simulink model "sobel_filter"  (Simulink 7.9)
settings: Solver=ode45  StartTime=0.0  StopTime=180*320  RelTol=1e-3
undefined symbols (not defined in the file): gray
libraries: xbsIndex_r4 x48, dspsigattribs x5, visionsinks x3, visiongeotforms x3, visionsources x1
settings Model: Creator=COMPUTER  LastModifiedBy=COMPUTER

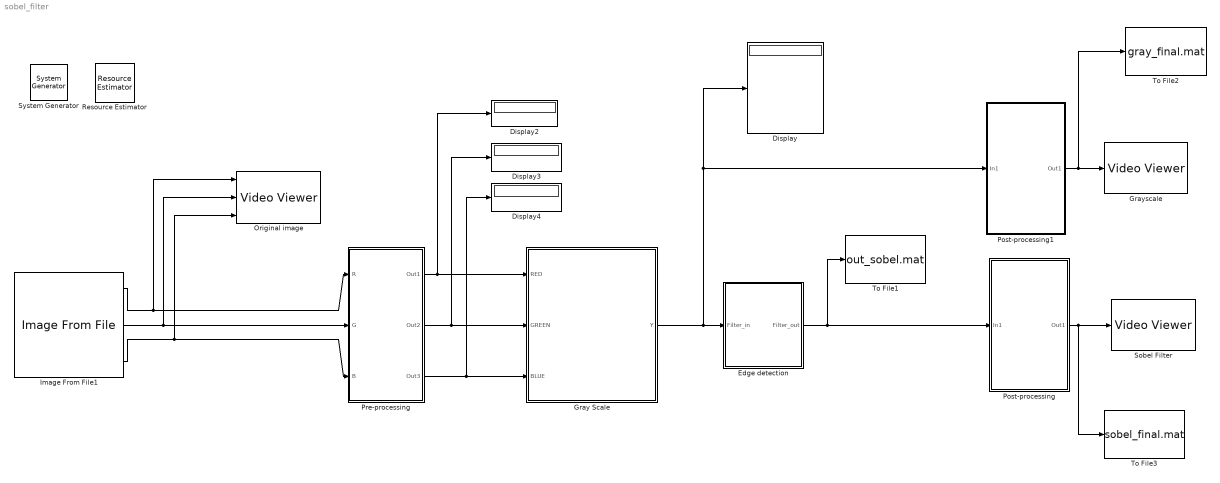
== system sobel_filter ==
  " System Generator" : xbsIndex_r4/ System Generator  Tag=genX  xilinxfamily=kintex7  part=xc7k325t  speed=-3  package=fbg676  synthesis_tool=XST  clock_wrapper=Clock Enables  directory=D:/DOAN1/Gray_conversion/ISE_software  proj_type=Project Navigator  Synth_file=XST Defaults  Impl_file=ISE Defaults  testbench=on  simulink_period=1  sysclk_period=10  dcm_input_clock_period=10  incr_netlist=off  trim_vbits=Everywhere in SubSystem  dbl_ovrd=According to Block Masks  core_generation=According to Block Masks  run_coregen=off  deprecated_control=off  eval_field=0  block_type=sysgen
  Display{,2..4} (4 alike) : Display
  Edge detection : Subsystem
  Gray Scale : Subsystem
  Grayscale : visionsinks/Video Viewer  inputType=Obsolete7b  imagePorts=One multidimensional signal  useColorMap=off  colormapValue=gray(256)  specRange=off  minInputVal=0  maxInputVal=255  FigPos=[2 1039 958 398]  AxisZoom=on  trueSizedOnce=off  OpenAtMdlStart=on
  Image From File1 : visionsources/Image From File  Tag=vipblks_nd  FileName=D:\DOAN1\Gray_conversion\hardware\straight_line_180_320.jpg  imagePorts=Separate color signals  Ts=inf  ImageDataType=uint8  Signed=on  WordLength=16  sdImageDataType=uint(8)  FractionLengthMode=User-defined  FractionLength=15  OutPortLabels=R|G|B
  Original image : visionsinks/Video Viewer  inputType=Obsolete7b  imagePorts=Separate color signals  useColorMap=off  colormapValue=gray(256)  specRange=off  minInputVal=0  maxInputVal=255  FigPos=[454 877 829 440]  AxisZoom=on  trueSizedOnce=off  OpenAtMdlStart=on
  Post-processing : Subsystem
  Post-processing1 : Subsystem
  Pre-processing : Subsystem
  Resource Estimator : xbsIndex_r4/Resource Estimator  Tag=resEstTag  Slices=0  FFs=0  BRAMs=0  LUTs=0  IOBs=0  EBMs=0  TBUFs=0  xl_use_estimator_area=off  est_options=Estimate  block_type=resource_estimator
      settings: AttributesFormatString=Resource\nEstimator
  Sobel Filter : visionsinks/Video Viewer  inputType=Obsolete7b  imagePorts=One multidimensional signal  useColorMap=off  colormapValue=gray(256)  specRange=off  minInputVal=0  maxInputVal=255  FigPos=[962 1039 958 919]  AxisZoom=on  trueSizedOnce=off  OpenAtMdlStart=on
  To File1 : ToFile  Filename=out_sobel.mat  MatrixName=sobel
  To File2 : ToFile  Filename=gray_final.mat  MatrixName=gray_final  SaveFormat=Timeseries
  To File3 : ToFile  Filename=sobel_final.mat  MatrixName=sobel_final  SaveFormat=Timeseries
  wires:
  Edge detection/1(Filter_out) -> Post-processing/1(In1), To File1/1
  Post-processing/1(Out1) -> Sobel Filter/1, To File3/1
  Pre-processing/1(Out1) -> Gray Scale/1(RED), Display2/1
  Image From File1/1 -> Original image/1, Pre-processing/1(R)
  Pre-processing/2(Out2) -> Gray Scale/2(GREEN), Display3/1
  Image From File1/2 -> Original image/2, Pre-processing/2(G)
  Pre-processing/3(Out3) -> Gray Scale/3(BLUE), Display4/1
  Image From File1/3 -> Original image/3, Pre-processing/3(B)
  Gray Scale/1(Y) -> Edge detection/1(Filter_in), Post-processing1/1(In1), Display/1
  Post-processing1/1(Out1) -> Grayscale/1, To File2/1

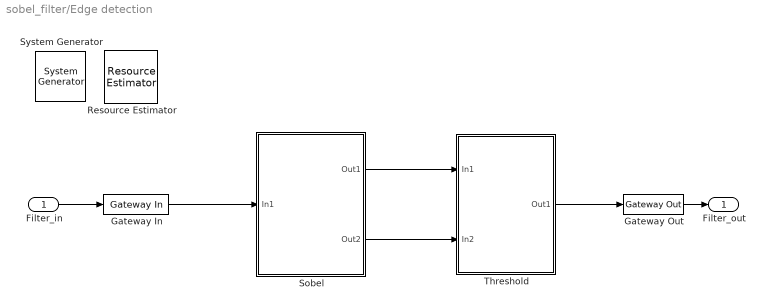
== system sobel_filter/Edge detection ==
  Filter_in : Inport
  " System Generator" : xbsIndex_r4/ System Generator  Tag=genX  xilinxfamily=kintex7  part=xc7k325t  speed=-3  package=fbg676  synthesis_tool=XST  clock_wrapper=Clock Enables  directory=./netlist  proj_type=Project Navigator  Synth_file=XST Defaults  Impl_file=ISE Defaults  testbench=off  simulink_period=1  sysclk_period=1.000000e+01  dcm_input_clock_period=10  incr_netlist=off  trim_vbits=Everywhere in SubSystem  dbl_ovrd=According to Block Masks  core_generation=According to Block Masks  run_coregen=off  deprecated_control=off  eval_field=0  block_type=sysgen
  Gateway In : xbsIndex_r4/Gateway In  gui_display_data_type=Fixed-point  arith_type=Unsigned  n_bits=8  bin_pt=0  preci_type=Single  exp_width=8  frac_width=24  quantization="Round  (unbiased: +/- Inf)"  overflow=Saturate  period=1  dbl_ovrd=off  timing_constraint=None  locs_specified=off  LOCs={}  UseAsADC=off  ADCChannel='1'  inherit_from_input=off  hdl_port=on  block_type=gatewayin
  Gateway Out : xbsIndex_r4/Gateway Out  inherit_from_input=off  hdl_port=on  timing_constraint="Data Rate;  Set 'FAST' Attribute"  locs_specified=off  LOCs={}  UseAsDAC=off  DACChannel='1'  block_type=gatewayout
  Resource Estimator : xbsIndex_r4/Resource Estimator  Tag=resEstTag  Slices=0  FFs=0  BRAMs=0  LUTs=0  IOBs=0  EBMs=0  TBUFs=0  xl_use_estimator_area=off  est_options=Estimate  block_type=resource_estimator
      settings: AttributesFormatString=Resource\nEstimator
  Sobel : Subsystem
  Threshold : Subsystem
  Filter_out : Outport
  wires:
  Filter_in/1 -> Gateway In/1
  Gateway Out/1 -> Filter_out/1
  Gateway In/1 -> Sobel/1(In1)
  Threshold/1(Out1) -> Gateway Out/1
  Sobel/1(Out1) -> Threshold/1(In1)
  Sobel/2(Out2) -> Threshold/2(In2)

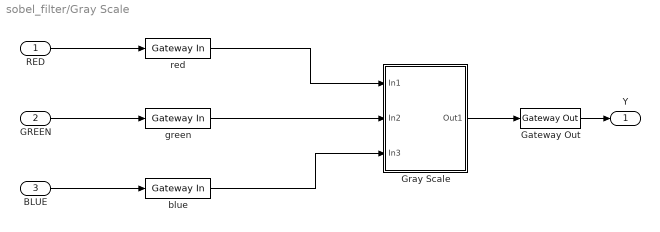
== system sobel_filter/Gray Scale ==
  RED : Inport
  GREEN : Inport  Port=2
  BLUE : Inport  Port=3
  Gateway Out : xbsIndex_r4/Gateway Out  inherit_from_input=off  hdl_port=on  timing_constraint="Data Rate;  Set 'FAST' Attribute"  locs_specified=off  LOCs={}  UseAsDAC=off  DACChannel='1'  block_type=gatewayout
  Gray Scale : Subsystem
  blue : xbsIndex_r4/Gateway In  gui_display_data_type=Fixed-point  arith_type="Signed  (2's comp)"  n_bits=8  bin_pt=0  preci_type=Single  exp_width=8  frac_width=24  quantization="Round  (unbiased: +/- Inf)"  overflow=Saturate  period=1  dbl_ovrd=off  timing_constraint=None  locs_specified=off  LOCs={}  UseAsADC=off  ADCChannel='1'  inherit_from_input=off  hdl_port=on  block_type=gatewayin
  green : xbsIndex_r4/Gateway In  gui_display_data_type=Fixed-point  arith_type="Signed  (2's comp)"  n_bits=8  bin_pt=0  preci_type=Single  exp_width=8  frac_width=24  quantization="Round  (unbiased: +/- Inf)"  overflow=Saturate  period=1  dbl_ovrd=off  timing_constraint=None  locs_specified=off  LOCs={}  UseAsADC=off  ADCChannel='1'  inherit_from_input=off  hdl_port=on  block_type=gatewayin
  red : xbsIndex_r4/Gateway In  gui_display_data_type=Fixed-point  arith_type=Unsigned  n_bits=8  bin_pt=0  preci_type=Single  exp_width=8  frac_width=24  quantization="Round  (unbiased: +/- Inf)"  overflow=Saturate  period=1  dbl_ovrd=off  timing_constraint=None  locs_specified=off  LOCs={}  UseAsADC=off  ADCChannel='1'  inherit_from_input=off  hdl_port=on  block_type=gatewayin
  Y : Outport
  wires:
  RED/1 -> red/1
  GREEN/1 -> green/1
  BLUE/1 -> blue/1
  Gateway Out/1 -> Y/1
  Gray Scale/1(Out1) -> Gateway Out/1
  red/1 -> Gray Scale/1(In1)
  green/1 -> Gray Scale/2(In2)
  blue/1 -> Gray Scale/3(In3)

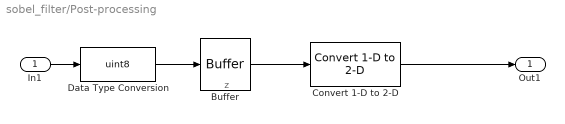
== system sobel_filter/Post-processing ==
  note: z
  In1 : Inport
  Buffer : Buffer  N=180*320
  Convert 1-D to 2-D : dspsigattribs/Convert 1-D to 2-D  M=180  N=320  frameBasedOut=off
  Data Type Conversion : DataTypeConversion  OutDataTypeStr=uint8  RndMeth=Round
  Out1 : Outport
  wires:
  Buffer/1 -> Convert 1-D to 2-D/1
  Convert 1-D to 2-D/1 -> Out1/1
  In1/1 -> Data Type Conversion/1
  Data Type Conversion/1 -> Buffer/1

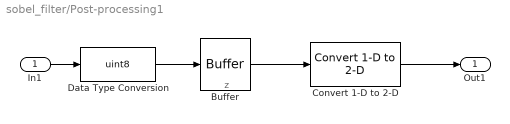
== system sobel_filter/Post-processing1 ==
  note: z
  In1 : Inport
  Buffer : Buffer  N=180*320
  Convert 1-D to 2-D : dspsigattribs/Convert 1-D to 2-D  M=180  N=320  frameBasedOut=off
  Data Type Conversion : DataTypeConversion  OutDataTypeStr=uint8
  Out1 : Outport
  wires:
  Buffer/1 -> Convert 1-D to 2-D/1
  Convert 1-D to 2-D/1 -> Out1/1
  In1/1 -> Data Type Conversion/1
  Data Type Conversion/1 -> Buffer/1

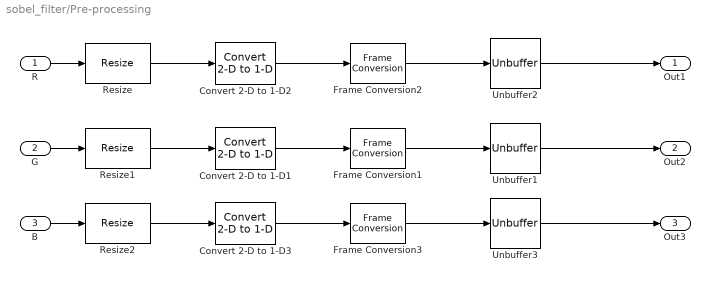
== system sobel_filter/Pre-processing ==
  R : Inport
  G : Inport  Port=2
  B : Inport  Port=3
  Convert 2-D to 1-D1 : dspsigattribs/Convert 2-D to 1-D
  Convert 2-D to 1-D2 : dspsigattribs/Convert 2-D to 1-D
  Convert 2-D to 1-D3 : dspsigattribs/Convert 2-D to 1-D
  Frame Conversion1 : FrameConversion
  Frame Conversion2 : FrameConversion
  Frame Conversion3 : FrameConversion
  Resize : visiongeotforms/Resize  specify=Number of output rows and columns  rfactor=[128 128]  outCols=25  outRows=25  outRowsCols=[180 320]  interp_method=Bilinear  antialias=on  useROI=off  roiFlag=off  prodOutputMode=Binary point scaling  prodOutputWordLength=32  prodOutputFracLength=10  roundingMode=Nearest  overflowMode=on
  Resize1 : visiongeotforms/Resize  specify=Number of output rows and columns  rfactor=[128 128]  outCols=25  outRows=25  outRowsCols=[180 320]  interp_method=Bilinear  antialias=on  useROI=off  roiFlag=off  prodOutputMode=Binary point scaling  prodOutputWordLength=32  prodOutputFracLength=10  roundingMode=Round  overflowMode=on
  Resize2 : visiongeotforms/Resize  specify=Number of output rows and columns  rfactor=[128 128]  outCols=25  outRows=25  outRowsCols=[180 320]  interp_method=Bilinear  antialias=on  useROI=off  roiFlag=off  prodOutputMode=Binary point scaling  prodOutputWordLength=32  prodOutputFracLength=10  roundingMode=Round  overflowMode=on
  Unbuffer1 : Unbuffer  SampleBasedProcessing=Same as frame based
  Unbuffer2 : Unbuffer  SampleBasedProcessing=Same as frame based
  Unbuffer3 : Unbuffer  SampleBasedProcessing=Same as frame based
  Out1 : Outport
  Out2 : Outport  Port=2
  Out3 : Outport  Port=3
  wires:
  Convert 2-D to 1-D2/1 -> Frame Conversion2/1
  Frame Conversion2/1 -> Unbuffer2/1
  Resize/1 -> Convert 2-D to 1-D2/1
  Convert 2-D to 1-D1/1 -> Frame Conversion1/1
  Frame Conversion1/1 -> Unbuffer1/1
  Resize1/1 -> Convert 2-D to 1-D1/1
  Convert 2-D to 1-D3/1 -> Frame Conversion3/1
  Frame Conversion3/1 -> Unbuffer3/1
  Resize2/1 -> Convert 2-D to 1-D3/1
  G/1 -> Resize1/1
  B/1 -> Resize2/1
  Unbuffer2/1 -> Out1/1
  Unbuffer1/1 -> Out2/1
  Unbuffer3/1 -> Out3/1
  R/1 -> Resize/1

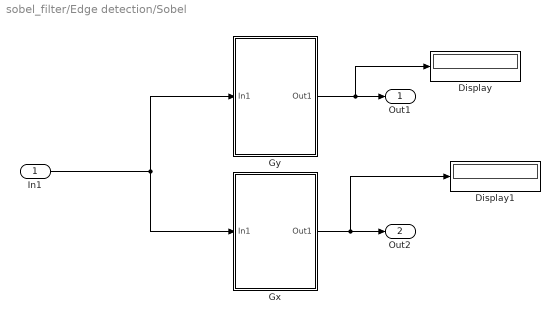
== system sobel_filter/Edge detection/Sobel ==
  In1 : Inport
  Display : Display
  Display1 : Display
  Gx : Subsystem
  Gy : Subsystem
  Out1 : Outport
  Out2 : Outport  Port=2
  wires:
  In1/1 -> Gx/1(In1), Gy/1(In1)
  Gy/1(Out1) -> Out1/1, Display/1
  Gx/1(Out1) -> Out2/1, Display1/1

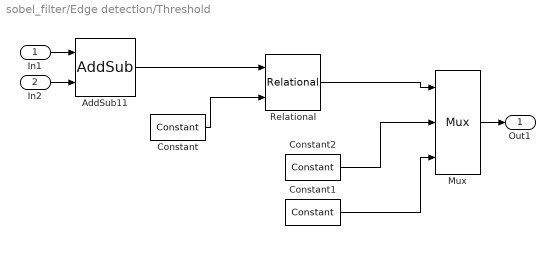
== system sobel_filter/Edge detection/Threshold ==
  In1 : Inport
  In2 : Inport  Port=2
  AddSub11 : xbsIndex_r4/AddSub  mode=Addition  use_carryin=off  use_carryout=off  en=off  latency=1  precision=Full  arith_type=Unsigned  n_bits=8  bin_pt=7  quantization=Truncate  overflow=Wrap  dbl_ovrd=off  use_behavioral_HDL=off  hw_selection=Fabric  pipelined=off  block_type=addsub
  Constant : xbsIndex_r4/Constant  const=200  gui_display_data_type=Fixed-point  arith_type=Unsigned  n_bits=8  bin_pt=0  preci_type=Single  exp_width=8  frac_width=24  explicit_period=off  period=1  equ=P=C  opselect=C  inp2=PCIN>>17  opr=+  inp1=P  carry=CIN  dbl_ovrd=off  block_type=constant
  Constant1 : xbsIndex_r4/Constant  const=255  gui_display_data_type=Floating-point  arith_type=Floating-point  n_bits=16  bin_pt=0  preci_type=Single  exp_width=8  frac_width=24  explicit_period=off  period=1  equ=P=C  opselect=C  inp2=PCIN>>17  opr=+  inp1=P  carry=CIN  dbl_ovrd=off  block_type=constant
  Constant2 : xbsIndex_r4/Constant  const=0  gui_display_data_type=Floating-point  arith_type=Floating-point  n_bits=16  bin_pt=0  preci_type=Single  exp_width=8  frac_width=24  explicit_period=off  period=1  equ=P=C  opselect=C  inp2=PCIN>>17  opr=+  inp1=P  carry=CIN  dbl_ovrd=off  block_type=constant
  Mux : xbsIndex_r4/Mux  inputs=2  en=off  latency=0  precision=Full  arith_type=Unsigned  n_bits=16  bin_pt=14  quantization=Truncate  overflow=Wrap  dbl_ovrd=off  block_type=mux
  Relational : xbsIndex_r4/Relational  mode=a>b  en=off  latency=1  dbl_ovrd=off  block_type=relational
  Out1 : Outport
  wires:
  Constant/1 -> Relational/2
  Relational/1 -> Mux/1
  Constant2/1 -> Mux/2
  Constant1/1 -> Mux/3
  AddSub11/1 -> Relational/1
  In1/1 -> AddSub11/1
  In2/1 -> AddSub11/2
  Mux/1 -> Out1/1

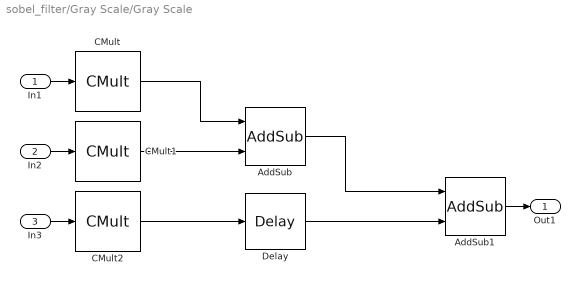
== system sobel_filter/Gray Scale/Gray Scale ==
  In1 : Inport
  In2 : Inport  Port=2
  In3 : Inport  Port=3
  AddSub : xbsIndex_r4/AddSub  mode=Addition  use_carryin=off  use_carryout=off  en=off  latency=0  precision=Full  arith_type=Unsigned  n_bits=8  bin_pt=7  quantization=Truncate  overflow=Wrap  dbl_ovrd=off  use_behavioral_HDL=off  hw_selection=Fabric  pipelined=off  block_type=addsub
  AddSub1 : xbsIndex_r4/AddSub  mode=Addition  use_carryin=off  use_carryout=off  en=off  latency=0  precision=Full  arith_type=Unsigned  n_bits=8  bin_pt=7  quantization=Truncate  overflow=Wrap  dbl_ovrd=off  use_behavioral_HDL=off  hw_selection=Fabric  pipelined=off  block_type=addsub
  CMult : xbsIndex_r4/CMult  const=0.299  gui_display_data_type=Fixed-point  const_n_bits=16  const_bin_pt=14  float_type=Custom  exp_bits=8  fraction_bits=24  en=off  latency=0  precision=Full  arith_type=Unsigned  n_bits=8  bin_pt=7  quantization=Truncate  overflow=Wrap  dbl_ovrd=off  use_behavioral_HDL=off  mem_type=Distributed RAM  pipeline=off  block_type=cmult
  CMult1 : xbsIndex_r4/CMult  const=0.587  gui_display_data_type=Fixed-point  const_n_bits=16  const_bin_pt=14  float_type=Custom  exp_bits=8  fraction_bits=24  en=off  latency=0  precision=Full  arith_type=Unsigned  n_bits=8  bin_pt=7  quantization=Truncate  overflow=Wrap  dbl_ovrd=off  use_behavioral_HDL=off  mem_type=Distributed RAM  pipeline=off  block_type=cmult
  CMult2 : xbsIndex_r4/CMult  const=0.114  gui_display_data_type=Fixed-point  const_n_bits=16  const_bin_pt=14  float_type=Custom  exp_bits=8  fraction_bits=24  en=off  latency=0  precision=Full  arith_type=Unsigned  n_bits=8  bin_pt=7  quantization=Truncate  overflow=Wrap  dbl_ovrd=off  use_behavioral_HDL=off  mem_type=Distributed RAM  pipeline=off  block_type=cmult
  Delay : xbsIndex_r4/Delay  rst=off  infoeditControl=Selection of Reset will increase slice count due to use of real FFs and instead of SRLs  en=off  latency=0  dbl_ovrd=off  reg_retiming=off  block_type=delay
  Out1 : Outport
  wires:
  CMult/1 -> AddSub/1
  CMult1/1 -> AddSub/2
  CMult2/1 -> Delay/1
  Delay/1 -> AddSub1/2
  AddSub/1 -> AddSub1/1
  In1/1 -> CMult/1
  In2/1 -> CMult1/1
  AddSub1/1 -> Out1/1
  In3/1 -> CMult2/1

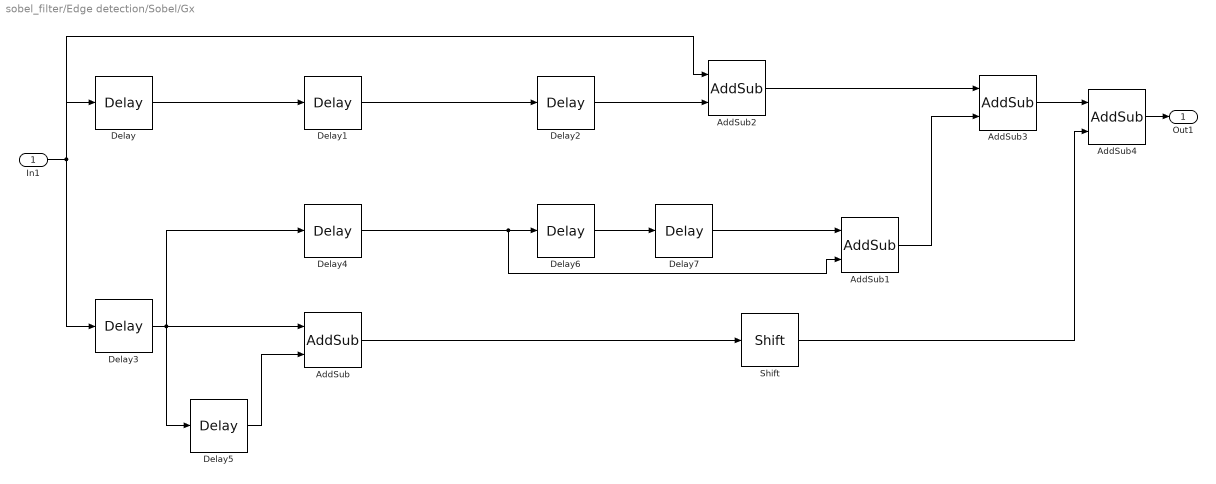
== system sobel_filter/Edge detection/Sobel/Gx ==
  In1 : Inport
  AddSub : xbsIndex_r4/AddSub  mode=Subtraction  use_carryin=off  use_carryout=off  en=off  latency=0  precision=Full  arith_type=Unsigned  n_bits=16  bin_pt=14  quantization=Truncate  overflow=Wrap  dbl_ovrd=off  use_behavioral_HDL=off  hw_selection=Fabric  pipelined=off  block_type=addsub
  AddSub1 : xbsIndex_r4/AddSub  mode=Subtraction  use_carryin=off  use_carryout=off  en=off  latency=0  precision=Full  arith_type=Unsigned  n_bits=16  bin_pt=14  quantization=Truncate  overflow=Wrap  dbl_ovrd=off  use_behavioral_HDL=off  hw_selection=Fabric  pipelined=off  block_type=addsub
  AddSub2 : xbsIndex_r4/AddSub  mode=Subtraction  use_carryin=off  use_carryout=off  en=off  latency=0  precision=Full  arith_type=Unsigned  n_bits=16  bin_pt=14  quantization=Truncate  overflow=Wrap  dbl_ovrd=off  use_behavioral_HDL=off  hw_selection=Fabric  pipelined=off  block_type=addsub
  AddSub3 : xbsIndex_r4/AddSub  mode=Addition  use_carryin=off  use_carryout=off  en=off  latency=0  precision=Full  arith_type=Unsigned  n_bits=16  bin_pt=14  quantization=Truncate  overflow=Wrap  dbl_ovrd=off  use_behavioral_HDL=off  hw_selection=Fabric  pipelined=off  block_type=addsub
  AddSub4 : xbsIndex_r4/AddSub  mode=Addition  use_carryin=off  use_carryout=off  en=off  latency=0  precision=Full  arith_type=Unsigned  n_bits=16  bin_pt=14  quantization=Truncate  overflow=Wrap  dbl_ovrd=off  use_behavioral_HDL=off  hw_selection=Fabric  pipelined=off  block_type=addsub
  Delay{,1..7} (8 alike) : xbsIndex_r4/Delay  rst=off  infoeditControl=Selection of Reset will increase slice count due to use of real FFs and instead of SRLs  en=off  latency=1  dbl_ovrd=off  reg_retiming=off  block_type=delay
  Shift : xbsIndex_r4/Shift  shift_dir=Left  shift_bits=1  en=off  latency=0  precision=Full  arith_type="Signed  (2's comp)"  n_bits=16  bin_pt=14  quantization=Truncate  overflow=Wrap  dbl_ovrd=off  block_type=shift
  Out1 : Outport
  wires:
  Delay/1 -> Delay1/1
  Delay1/1 -> Delay2/1
  Delay3/1 -> Delay4/1, AddSub/1, Delay5/1
  Delay5/1 -> AddSub/2
  AddSub/1 -> Shift/1
  Delay6/1 -> Delay7/1
  Delay4/1 -> Delay6/1, AddSub1/2
  Delay2/1 -> AddSub2/2
  AddSub2/1 -> AddSub3/1
  AddSub1/1 -> AddSub3/2
  AddSub3/1 -> AddSub4/1
  Shift/1 -> AddSub4/2
  Delay7/1 -> AddSub1/1
  In1/1 -> Delay3/1, AddSub2/1, Delay/1
  AddSub4/1 -> Out1/1

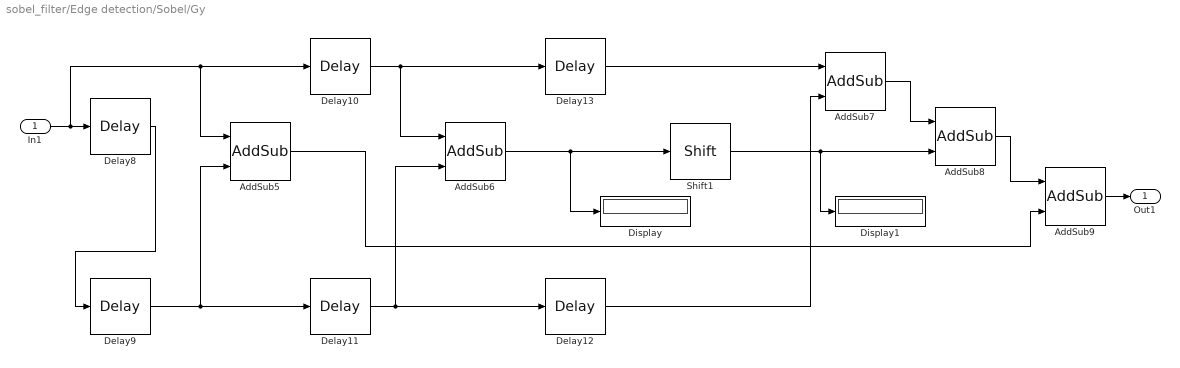
== system sobel_filter/Edge detection/Sobel/Gy ==
  In1 : Inport
  AddSub5 : xbsIndex_r4/AddSub  mode=Subtraction  use_carryin=off  use_carryout=off  en=off  latency=0  precision=Full  arith_type=Unsigned  n_bits=16  bin_pt=14  quantization=Truncate  overflow=Wrap  dbl_ovrd=off  use_behavioral_HDL=off  hw_selection=Fabric  pipelined=off  block_type=addsub
  AddSub6 : xbsIndex_r4/AddSub  mode=Subtraction  use_carryin=off  use_carryout=off  en=off  latency=0  precision=Full  arith_type=Unsigned  n_bits=16  bin_pt=14  quantization=Truncate  overflow=Wrap  dbl_ovrd=off  use_behavioral_HDL=off  hw_selection=Fabric  pipelined=off  block_type=addsub
  AddSub7 : xbsIndex_r4/AddSub  mode=Subtraction  use_carryin=off  use_carryout=off  en=off  latency=0  precision=Full  arith_type=Unsigned  n_bits=16  bin_pt=14  quantization=Truncate  overflow=Wrap  dbl_ovrd=off  use_behavioral_HDL=off  hw_selection=Fabric  pipelined=off  block_type=addsub
  AddSub8 : xbsIndex_r4/AddSub  mode=Addition  use_carryin=off  use_carryout=off  en=off  latency=0  precision=Full  arith_type=Unsigned  n_bits=16  bin_pt=14  quantization=Truncate  overflow=Wrap  dbl_ovrd=off  use_behavioral_HDL=off  hw_selection=Fabric  pipelined=off  block_type=addsub
  AddSub9 : xbsIndex_r4/AddSub  mode=Addition  use_carryin=off  use_carryout=off  en=off  latency=0  precision=Full  arith_type=Unsigned  n_bits=16  bin_pt=14  quantization=Truncate  overflow=Wrap  dbl_ovrd=off  use_behavioral_HDL=off  hw_selection=Fabric  pipelined=off  block_type=addsub
  Delay{8..13} (6 alike) : xbsIndex_r4/Delay  rst=off  infoeditControl=Selection of Reset will increase slice count due to use of real FFs and instead of SRLs  en=off  latency=1  dbl_ovrd=off  reg_retiming=off  block_type=delay
  Display : Display
  Display1 : Display
  Shift1 : xbsIndex_r4/Shift  shift_dir=Left  shift_bits=1  en=off  latency=0  precision=Full  arith_type="Signed  (2's comp)"  n_bits=16  bin_pt=14  quantization=Truncate  overflow=Wrap  dbl_ovrd=off  block_type=shift
  Out1 : Outport
  wires:
  Delay8/1 -> Delay9/1
  Delay9/1 -> AddSub5/2, Delay11/1
  Delay10/1 -> AddSub6/1, Delay13/1
  Delay11/1 -> AddSub6/2, Delay12/1
  AddSub6/1 -> Shift1/1, Display/1
  Delay13/1 -> AddSub7/1
  Delay12/1 -> AddSub7/2
  AddSub7/1 -> AddSub8/1
  Shift1/1 -> AddSub8/2, Display1/1
  AddSub8/1 -> AddSub9/1
  AddSub5/1 -> AddSub9/2
  In1/1 -> AddSub5/1, Delay10/1, Delay8/1
  AddSub9/1 -> Out1/1
